simulink model "wifi_spreading"  (R2021a)
settings: Solver=VariableStepDiscrete  StartTime=0.0  StopTime=160e-6  RelTol=1e-3
libraries: commseqgen3 x3, dspsrcs4 x2, commchan3 x1, commfilt2 x1, commutil2 x1
settings Model: Creator=Tomas  LastModifiedBy=Tomas

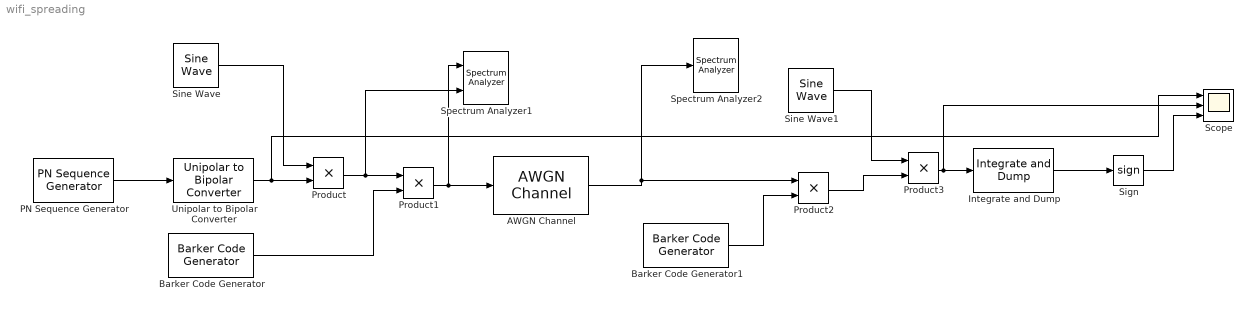
== system wifi_spreading ==
  AWGN Channel : commchan3/AWGN Channel  InputProcessing=Columns as channels (frame based)  seed=67  noiseMode=Variance from mask  EbNodB=10  EsNodB=10  SNRdB=100  bitsPerSym=1  Ps=1  Tsym=1  variance=1000
  Barker Code Generator : commseqgen3/Barker Code Generator  Length=7  LengthSimulink=11  SampleTime=1/11e6  SamplesPerFrame=1  OutputDataType=double  SimulateUsing=Code generation
      settings: SourceProductBaseCode=CM
  Barker Code Generator1 : commseqgen3/Barker Code Generator  Length=7  LengthSimulink=11  SampleTime=1/11e6  SamplesPerFrame=1  OutputDataType=double  SimulateUsing=Code generation
      settings: SourceProductBaseCode=CM
  Integrate and Dump : commfilt2/Integrate and Dump  obssamples=10000  offsetsamples=0  nodump=off  roundingMode=Floor  overflowMode=off  outputDataTypeStr=Inherit: Same as accumulator  outputLastDataTypeStr=Inherit: Same as accumulator
  PN Sequence Generator : commseqgen3/PN Sequence Generator  poly='z^7+z^6 + 1'  ini_sta=[1 1 1 1 1 1 1]  outBitMaskSource=Dialog parameter  shift=0  outVarSiz=off  maxOutSizeMode=Dialog parameter  maxOutSize=[10 1]  Ts=1/1e6  sampPerFrame=1  reset=off  bitPackedOutputs=off  outDataType=double  numPackedBits=8  bitPackDataSigned=off  bitPackedOutDType=double
  Product{,1..3} (4 alike) : Product  SampleTime=0.1e-9
  Scope : Scope  NumInputPorts=3
  Sign : Signum
  Sine Wave : dspsrcs4/Sine Wave  Amplitude=1  Frequency=200e6  Phase=0  SampleMode=Discrete  OutComplex=Real  CompMethod=Trigonometric fcn  TableSize=Speed  SampleTime=1/1e10  SamplesPerFrame=1  ResetState=Restart at time zero  OutputFrames=off  dataType=double  wordLen=16  udDataType=sfix(16)  fracBitsMode=Best precision  numFracBits=15  OutDataTypeStr=double  LastOutDataTypeStr=double
  Sine Wave1 : dspsrcs4/Sine Wave  Amplitude=1  Frequency=200e6  Phase=0  SampleMode=Discrete  OutComplex=Real  CompMethod=Trigonometric fcn  TableSize=Speed  SampleTime=1/1e10  SamplesPerFrame=1  ResetState=Restart at time zero  OutputFrames=off  dataType=double  wordLen=16  udDataType=sfix(16)  fracBitsMode=Best precision  numFracBits=15  OutDataTypeStr=double  LastOutDataTypeStr=double
  Spectrum Analyzer1 : SpectrumAnalyzer  NumInputPorts=2
  Spectrum Analyzer2 : SpectrumAnalyzer
  Unipolar to Bipolar Converter : commutil2/Unipolar to Bipolar Converter  M=2  polarity=Positive  dataType=Inherit via internal rule
  wires:
  PN Sequence Generator/1 -> Unipolar to Bipolar Converter/1
  Product1/1 -> AWGN Channel/1, Spectrum Analyzer1/1
  Sine Wave/1 -> Product/1
  Unipolar to Bipolar Converter/1 -> Scope/1, Product/2
  Product/1 -> Spectrum Analyzer1/2, Product1/1
  Barker Code Generator/1 -> Product1/2
  AWGN Channel/1 -> Product2/1, Spectrum Analyzer2/1
  Barker Code Generator1/1 -> Product2/2
  Product2/1 -> Product3/2
  Sine Wave1/1 -> Product3/1
  Integrate and Dump/1 -> Sign/1
  Sign/1 -> Scope/3
  Product3/1 -> Scope/2, Integrate and Dump/1
